simulink model "AB_switchtime_spline_real_time"  (R2025a)
settings: Solver=ode4  StartTime=0.0  StopTime=inf  FixedStep=1/500  RelTol=1e-3  EnableMultiTasking=on
InitFcn:
  | home = [0.45; 0; 0.49];
  | pick = [0.3; 0; 0.3];
  | place = [-0.25; -0.25; 0.01];
  | waypoints = ...
  | [pick, pick,place ,place ,home]' ;
undefined symbols (not defined in the file or in its folder): HIL, qc_get_step_size
libraries: quarc_library x19, simulink x2
(part 2 of 2)

== matlab function AB_switchtime_spline_real_time/objective position ==
  data: p input; gamma input; phi_optimal output; phi_prev input
function phi_optimal = qarmInverseKinematics_target(p, gamma, phi_prev)
%% QARM Inverse Kinematics (NaN-safe, limite saturée + workspace check)
% p        : position [x;y;z] en m
% gamma    : rotation poignet (rad)
% phi_prev : configuration précédente [4x1] en rad
% phi_optimal : configuration atteignable [4x1] rad

%% Paramètres du manipulateur
L1 = 0.1400; L2 = 0.3500; L3 = 0.0500; L4 = 0.2500; L5 = 0.1500;
beta = atan(L3/L2);
lambda1 = L1;
lambda2 = sqrt(L2^2 + L3^2);
lambda3 = L4 + L5;

%% Initialisation
theta = zeros(4,4);
phi   = zeros(4,4);

%% --- Calcul theta2 / theta3 ---
A = lambda2; 
C = -lambda3; 
H = lambda1 - p(3);

D1 = -sqrt(p(1)^2 + p(2)^2); 
D2 =  sqrt(p(1)^2 + p(2)^2);

F1 = (D1^2 + H^2 - A^2 - C^2)/(2*A);
F2 = (D2^2 + H^2 - A^2 - C^2)/(2*A);

% Solutions 1/2
if C^2 - F1^2 < 0
    warning('Position non atteignable pour solution 1/2 : saturation');
    theta(3,1) = sign(C)*pi/2;  
    theta(3,2) = sign(C)*pi/2;
else
    theta(3,1) = 2*atan2( C + sqrt(C^2 - F1^2), F1 );
    theta(3,2) = 2*atan2( C - sqrt(C^2 - F1^2), F1 );
end

% Solutions 3/4
if C^2 - F2^2 < 0
    warning('Position non atteignable pour solution 3/4 : saturation');
    theta(3,3) = sign(C)*pi/2;
    theta(3,4) = sign(C)*pi/2;
else
    theta(3,3) = 2*atan2( C + sqrt(C^2 - F2^2), F2 );
    theta(3,4) = 2*atan2( C - sqrt(C^2 - F2^2), F2 );
end

%% --- Calcul theta2 ---
for i = 1:4
    D = D1; 
    if i > 2
        D = D2;
    end
    M = A + C*sin(theta(3,i));
    N = -C*cos(theta(3,i));
    if abs(M) < 1e-6
        M = sign(M)*1e-6;
    end
    cos_term = (D*M + H*N)/(M^2 + N^2);
    sin_term = (H - N*cos_term)/M;
    theta(2,i) = atan2(sin_term, cos_term);
end

%% --- Calcul theta1 ---
for i = 1:4
    denom = lambda2*cos(theta(2,i)) - lambda3*sin(theta(2,i)+theta(3,i));
    if abs(denom) < 1e-6
        denom = sign(denom)*1e-6;
    end
    theta(1,i) = atan2(p(2)/denom, p(1)/denom);
end

%% --- Remap vers angles QARM ---
phi(1,:) = theta(1,:);
phi(2,:) = theta(2,:) - beta + pi/2;
phi(3,:) = theta(3,:) + beta;
phi(4,:) = gamma;
phi = mod(phi+pi, 2*pi) - pi; % normalisation [-pi,pi]

%% --- Saturation des limites articulaires ---
for i = 1:4
    phi(:,i) = saturate_joint_limits(phi(:,i));
end

%% --- Choix solution la plus proche de phi_prev dans le workspace ---
phi_optimal = phi_prev;     % par défaut: on reste où on est
best_norm   = inf;

for i = 1:4
    if ~isInsideWorkspace(phi(:,i))
        continue;           % solution rejetée: hors workspace
    end

    current_norm = norm(phi(:,i) - phi_prev);
    if current_norm < best_norm
        phi_optimal = phi(:,i);
        best_norm   = current_norm;
    end
end

if isinf(best_norm)
    warning('Aucune solution IK dans le workspace. On garde phi_prev.');
    phi_optimal = phi_prev;
end

end

%% --- Fonction de saturation ---
function phi_sat = saturate_joint_limits(phi)
limits = [
    -170  170;
    -80    80;
    -95    75;
    -160  160
]*pi/180;
phi_sat = phi;
for i = 1:4
    if phi(i) < limits(i,1), phi_sat(i) = limits(i,1); end
    if phi(i) > limits(i,2), phi_sat(i) = limits(i,2); end
end
end

%% --- Test de workspace via cinématique directe ---
function inside = isInsideWorkspace(phi)
    % Paramètres de l'enveloppe
    rMax = 0.8 * 0.78;      % rayon maximal autorisé (à ajuster)

    % Robot persistant pour la FK
    persistent robot eeName
    if isempty(robot)
        robot = loadrobot("quanserQArm", DataFormat="row");
        eeName = robot.BodyNames{end};
    end

    % Cinématique directe
    T = getTransform(robot, phi', eeName);   % phi' = row vector
    p = tform2trvec(T);                     % [x y z]

    x = p(1); y = p(2); z = p(3);
    r = norm(p);

    % 1) dedans la sphère
    % 2) pas dans le quadrant x<0 & z<0
    inside = (r < rMax) && ~((x < 0) && (z < 0));
end

== matlab function AB_switchtime_spline_real_time/Time_computation ==
  data: q0 input; T_min output size=1; q_end input
function T_min = T_min (q0, q_end)
    v_max = deg2rad([90 90 90 90]);
    T_vector = abs(q_end - q0) ./ v_max;
    T_min = max(T_vector(:)) * 1.2;
   
end

== matlab function AB_switchtime_spline_real_time/is_the_target_changed?1 ==
  data: p_obj input; final_p_obj output
function final_p_obj  = out_of_target(p_obj)
    eps_val = 1e-6;
    R_max = 0.7;

    norm_p = norm(p_obj);
    
    if norm_p > R_max
        final_p_obj = R_max * (p_obj / (norm_p + eps_val));
    else
        final_p_obj = p_obj;
    end
    
end

== matlab function AB_switchtime_spline_real_time/forward kinematics1 ==
  data: p3 output; R03 output; phi input; p4 output; R04 output; p_cam_0 output; p_obj_0 output; p_obj_cam input
function [p3, R03, p4, R04, p_cam_0,p_obj_0] = qarmForwardKinematics_target(phi,p_obj_cam)

%% QUANSER_ARM_FPK
% v 4.0 - 4th June 2020

% REFERENCE: 
% Chapter 3. Forward Kinematics
% Robot Dynamics and Control 
% Spong, Vidyasagar
% 1989

% INPUTS:
% phi     : Alternate joint angles vector 4 x 1

% OUTPUTS:
% p4      : End-effector frame {4} position vector expressed in base frame {0}
% R04     : rotation matrix from end-effector frame {4} to base frame {0}

%% Manipulator parameters:
L1 = 0.1400;
L2 = 0.3500;
L3 = 0.0500;
L4 = 0.2500;
L5 = 0.1500;

%% Alternate parameters
l1 = L1;
l2 = sqrt(L2^2 + L3^2);
l3 = L4 + L5;
beta = atan(L3/L2);

%% From phi space to theta space 
theta = phi;
theta(1) = phi(1);
theta(2) = phi(2) + beta - pi/2;
theta(3) = phi(3) - beta;
theta(4) = phi(4);

%% Transformation matrices for all frames:

% T{i-1}{i} = quanser_arm_DH(  a, alpha,  d,     theta );
        T01 = quanser_arm_DH(  0, -pi/2, l1,  theta(1) );
        T12 = quanser_arm_DH( l2,     0,  0,  theta(2) );
        T23 = quanser_arm_DH(  0, -pi/2,  0,  theta(3) );
        T34 = quanser_arm_DH(  0,     0, l3,  theta(4) );

        T02 = T01*T12;
        T03 = T02*T23;
        T04 = T03*T34;

%% Position of end-effector Transformation

% Extract the Position vector 
% p1   = T01(1:3,4);
% p2   = T02(1:3,4);
p3   = T03(1:3,4);
p4   = T04(1:3,4);

% Extract the Rotation matrix
% R01 = T01(1:3,1:3);
% R02 = T02(1:3,1:3);
R03 = T03(1:3,1:3);
R04 = T04(1:3,1:3);

d_tilde = 0.3; % distance entre P03 et la caméra (m)

% position de la caméra dans le frame de l'articulation 3
p_cam_3 = [0; 0; d_tilde]; 

% position de la caméra dans le frame global {0}
p_cam_0 = p3 + R03 * p_cam_3;

R_cam_3 = [ -1  0  0;
             0  1  0;
             0  0 -1 ];  % exemple si on inverse X et Z

R_cam_3 = [ 0  -1  0;
             1 0  0;
             0  0 1 ];  % exemple si on inverse X et Z

R_cam_0 = R03 * R_cam_3;  % rotation de la caméra dans le global

p_obj_0 = p_cam_0 + R_cam_0 * p_obj_cam;


end

function T = quanser_arm_DH(a,alpha,d,theta)

%% QUANSER_ARM_DH
% v 1.0 - 26th March 2019

% REFERENCE: 
% Chapter 3. Forward and Inverse Kinematics
% Robot Modeling and Control 
% Spong, Hutchinson, Vidyasagar
% 2006

% INPUTS:
% a       :   translation  : along : x_{i}   : from : z_{i-1} : to : z_{i}
% alpha   :      rotation  : about : x_{i}   : from : z_{i-1} : to : z_{i}
% d       :   translation  : along : z_{i-1} : from : x_{i-1} : to : x_{i}
% theta   :      rotation  : about : z_{i-1} : from : x_{i-1} : to : x_{i}
% NOTE: Standard DH Parameters

% OUTPUTS:
% T       : transformation                   : from :     {i} : to : {i-1}

%%
% Rotation Transformation about z axis by theta
T_R_z = [cos(theta) -sin(theta) 0 0;
         sin(theta)  cos(theta) 0 0;
                  0           0 1 0;
                  0           0 0 1];
     
% Translation Transformation along z axis by d
T_T_z = [1 0 0 0;
         0 1 0 0;
         0 0 1 d;
         0 0 0 1];

% Translation Transformation along x axis by a
T_T_x = [1 0 0 a;
         0 1 0 0;
         0 0 1 0;
         0 0 0 1];

% Rotation Transformation about x axis by alpha
T_R_x = [1          0           0 0;
         0 cos(alpha) -sin(alpha) 0;
         0 sin(alpha)  cos(alpha) 0;
         0          0           0 1];

% For a transformation FROM frame {i} TO frame {i-1}: A
T = T_R_z*T_T_z*T_T_x*T_R_x;

end

== matlab function AB_switchtime_spline_real_time/is_the_target_changed? ==
  data: p_target input; newTarget output; time output
function [newTarget, time]= Target_changed(p_target)

    persistent p_prev
    persistent T
        if isempty(p_prev)
            p_prev = zeros(size(p_target));
        end

        if isempty(T)
            T = 0.01;
        end
    
        %distance p_target and p_prev
        dp = p_target - p_prev;
        norm_dp = norm(dp);
   
        threshold = 0.05;   % [m]
    
        if norm_dp > threshold
            newTarget = 1;
            p_prev = p_target;
            T = 0.01;

               
        else
            newTarget = 0;
            T = T+0.01;
            %we don't switch

        
            
        end 
        time = T;
    
        
end

== matlab function AB_switchtime_spline_real_time/forward kinematics ==
  data: phi input; p4 output; R04 output
function [p4, R04] = qarmForwardKinematics(phi)

%% QUANSER_ARM_FPK
% v 4.0 - 4th June 2020

% REFERENCE: 
% Chapter 3. Forward Kinematics
% Robot Dynamics and Control 
% Spong, Vidyasagar
% 1989

% INPUTS:
% phi     : Alternate joint angles vector 4 x 1

% OUTPUTS:
% p4      : End-effector frame {4} position vector expressed in base frame {0}
% R04     : rotation matrix from end-effector frame {4} to base frame {0}

%% Manipulator parameters:
L1 = 0.1400;
L2 = 0.3500;
L3 = 0.0500;
L4 = 0.2500;
L5 = 0.1500;

%% Alternate parameters
l1 = L1;
l2 = sqrt(L2^2 + L3^2);
l3 = L4 + L5;
beta = atan(L3/L2);

%% From phi space to theta space 
theta = phi;
theta(1) = phi(1);
theta(2) = phi(2) + beta - pi/2;
theta(3) = phi(3) - beta;
theta(4) = phi(4);

%% Transformation matrices for all frames:

% T{i-1}{i} = quanser_arm_DH(  a, alpha,  d,     theta );
        T01 = quanser_arm_DH(  0, -pi/2, l1,  theta(1) );
        T12 = quanser_arm_DH( l2,     0,  0,  theta(2) );
        T23 = quanser_arm_DH(  0, -pi/2,  0,  theta(3) );
        T34 = quanser_arm_DH(  0,     0, l3,  theta(4) );

        T02 = T01*T12;
        T03 = T02*T23;
        T04 = T03*T34;

%% Position of end-effector Transformation

% Extract the Position vector 
% p1   = T01(1:3,4);
% p2   = T02(1:3,4);
% p3   = T03(1:3,4);
p4   = T04(1:3,4);

% Extract the Rotation matrix
% R01 = T01(1:3,1:3);
% R02 = T02(1:3,1:3);
% R03 = T03(1:3,1:3);
R04 = T04(1:3,1:3);

end

function T = quanser_arm_DH(a,alpha,d,theta)

%% QUANSER_ARM_DH
% v 1.0 - 26th March 2019

% REFERENCE: 
% Chapter 3. Forward and Inverse Kinematics
% Robot Modeling and Control 
% Spong, Hutchinson, Vidyasagar
% 2006

% INPUTS:
% a       :   translation  : along : x_{i}   : from : z_{i-1} : to : z_{i}
% alpha   :      rotation  : about : x_{i}   : from : z_{i-1} : to : z_{i}
% d       :   translation  : along : z_{i-1} : from : x_{i-1} : to : x_{i}
% theta   :      rotation  : about : z_{i-1} : from : x_{i-1} : to : x_{i}
% NOTE: Standard DH Parameters

% OUTPUTS:
% T       : transformation                   : from :     {i} : to : {i-1}

%%
% Rotation Transformation about z axis by theta
T_R_z = [cos(theta) -sin(theta) 0 0;
         sin(theta)  cos(theta) 0 0;
                  0           0 1 0;
                  0           0 0 1];
     
% Translation Transformation along z axis by d
T_T_z = [1 0 0 0;
         0 1 0 0;
         0 0 1 d;
         0 0 0 1];

% Translation Transformation along x axis by a
T_T_x = [1 0 0 a;
         0 1 0 0;
         0 0 1 0;
         0 0 0 1];

% Rotation Transformation about x axis by alpha
T_R_x = [1          0           0 0;
         0 cos(alpha) -sin(alpha) 0;
         0 sin(alpha)  cos(alpha) 0;
         0          0           0 1];

% For a transformation FROM frame {i} TO frame {i-1}: A
T = T_R_z*T_T_z*T_T_x*T_R_x;

end

== matlab function AB_switchtime_spline_real_time/target_phi ==
  data: coeffs input; q output; t input
function q = evalCubic4(coeffs, t)
% coeffs: 4x4, righe = [a0;a1;a2;a3], colonne = giunti
% t: scalare
% q: 4x1

    a0 = coeffs(1, :).';  % 4x1
    a1 = coeffs(2, :).';
    a2 = coeffs(3, :).';
    a3 = coeffs(4, :).';

    q = a0 + a1*t + a2*(t^2) + a3*(t^3);
end

== matlab function AB_switchtime_spline_real_time/differential kinematics ==
  data: phi input; J output
function J   = qarmDifferentialKinematics(phi)

%% QUANSER_ARM_FDK
% v 1.0 - 13th August 2020

% REFERENCE: 
% Chapter 5. Velocity Kinematics
% Robot Dynamics and Control 
% Spong, Vidyasagar
% 1989

% INPUTS:
% phi     : Alternate joint angles vector 4 x 1

% OUTPUTS:
% p4      : End-effector frame {4} position vector expressed in base frame {0}
% R04     : rotation matrix from end-effector frame {4} to base frame {0}

%% Manipulator parameters:
L1 = 0.1400;
L2 = 0.3500;
L3 = 0.0500;
L4 = 0.2500;
L5 = 0.1500;

%% Alternate parameters
l1 = L1;
l2 = sqrt(L2^2 + L3^2);
l3 = L4 + L5;
beta = atan(L3/L2);

%% From phi space to theta space 
theta = phi;
theta(1) = phi(1);
theta(2) = phi(2) + beta - pi/2;
theta(3) = phi(3) - beta;
theta(4) = phi(4);

%% Precompute sines and cosines
c1 = cos(theta(1)); s1 = sin(theta(1));
c2 = cos(theta(2)); s2 = sin(theta(2));
c23 = cos(theta(2) + theta(3)); s23 = sin(theta(2) + theta(3));

%% Jacobian term definition:

J = eye(4);
J(1,1) = -l2 * s1 * c2 + l3 * s1 * s23;
J(1,2) = -l2 * c1 * s2 - l3 * c1 * c23;
J(1,3) = -l3 * c1 * c23;
J(1,4) = 0;

J(2,1) =  l2 * c1 * c2 - l3 * c1 * s23;
J(2,2) = -l2 * s1 * s2 - l3 * s1 * c23;
J(2,3) = -l3 * s1 * c23;
J(2,4) = 0;

J(3,1) =  0;
J(3,2) = -l2 * c2 + l3 * s23;
J(3,3) =  l3 * s23;
J(3,4) = 0;

J(4,1) =  0;
J(4,2) =  0;
J(4,3) =  0;
J(4,4) =  1;

end

== matlab function AB_switchtime_spline_real_time/forward kinematics - measurement ==
  data: phi input; p4 output; R04 output
function [p4, R04] = qarmForwardKinematics(phi)

%% QUANSER_ARM_FPK
% v 4.0 - 4th June 2020

% REFERENCE: 
% Chapter 3. Forward Kinematics
% Robot Dynamics and Control 
% Spong, Vidyasagar
% 1989

% INPUTS:
% phi     : Alternate joint angles vector 4 x 1

% OUTPUTS:
% p4      : End-effector frame {4} position vector expressed in base frame {0}
% R04     : rotation matrix from end-effector frame {4} to base frame {0}

%% Manipulator parameters:
L1 = 0.1400;
L2 = 0.3500;
L3 = 0.0500;
L4 = 0.2500;
L5 = 0.1500;

%% Alternate parameters
l1 = L1;
l2 = sqrt(L2^2 + L3^2);
l3 = L4 + L5;
beta = atan(L3/L2);

%% From phi space to theta space 
theta = phi;
theta(1) = phi(1);
theta(2) = phi(2) + beta - pi/2;
theta(3) = phi(3) - beta;
theta(4) = phi(4);

%% Transformation matrices for all frames:

% T{i-1}{i} = quanser_arm_DH(  a, alpha,  d,     theta );
        T01 = quanser_arm_DH(  0, -pi/2, l1,  theta(1) );
        T12 = quanser_arm_DH( l2,     0,  0,  theta(2) );
        T23 = quanser_arm_DH(  0, -pi/2,  0,  theta(3) );
        T34 = quanser_arm_DH(  0,     0, l3,  theta(4) );

        T02 = T01*T12;
        T03 = T02*T23;
        T04 = T03*T34;

%% Position of end-effector Transformation

% Extract the Position vector 
% p1   = T01(1:3,4);
% p2   = T02(1:3,4);
% p3   = T03(1:3,4);
p4   = T04(1:3,4);

% Extract the Rotation matrix
% R01 = T01(1:3,1:3);
% R02 = T02(1:3,1:3);
% R03 = T03(1:3,1:3);
R04 = T04(1:3,1:3);

end

function T = quanser_arm_DH(a,alpha,d,theta)

%% QUANSER_ARM_DH
% v 1.0 - 26th March 2019

% REFERENCE: 
% Chapter 3. Forward and Inverse Kinematics
% Robot Modeling and Control 
% Spong, Hutchinson, Vidyasagar
% 2006

% INPUTS:
% a       :   translation  : along : x_{i}   : from : z_{i-1} : to : z_{i}
% alpha   :      rotation  : about : x_{i}   : from : z_{i-1} : to : z_{i}
% d       :   translation  : along : z_{i-1} : from : x_{i-1} : to : x_{i}
% theta   :      rotation  : about : z_{i-1} : from : x_{i-1} : to : x_{i}
% NOTE: Standard DH Parameters

% OUTPUTS:
% T       : transformation                   : from :     {i} : to : {i-1}

%%
% Rotation Transformation about z axis by theta
T_R_z = [cos(theta) -sin(theta) 0 0;
         sin(theta)  cos(theta) 0 0;
                  0           0 1 0;
                  0           0 0 1];
     
% Translation Transformation along z axis by d
T_T_z = [1 0 0 0;
         0 1 0 0;
         0 0 1 d;
         0 0 0 1];

% Translation Transformation along x axis by a
T_T_x = [1 0 0 a;
         0 1 0 0;
         0 0 1 0;
         0 0 0 1];

% Rotation Transformation about x axis by alpha
T_R_x = [1          0           0 0;
         0 cos(alpha) -sin(alpha) 0;
         0 sin(alpha)  cos(alpha) 0;
         0          0           0 1];

% For a transformation FROM frame {i} TO frame {i-1}: A
T = T_R_z*T_T_z*T_T_x*T_R_x;

end

== matlab function AB_switchtime_spline_real_time/forward kinematics3 ==
  data: phi input; p4 output; R04 output
function [p4, R04] = qarmForwardKinematics(phi)

%% QUANSER_ARM_FPK
% v 4.0 - 4th June 2020

% REFERENCE: 
% Chapter 3. Forward Kinematics
% Robot Dynamics and Control 
% Spong, Vidyasagar
% 1989

% INPUTS:
% phi     : Alternate joint angles vector 4 x 1

% OUTPUTS:
% p4      : End-effector frame {4} position vector expressed in base frame {0}
% R04     : rotation matrix from end-effector frame {4} to base frame {0}

%% Manipulator parameters:
L1 = 0.1400;
L2 = 0.3500;
L3 = 0.0500;
L4 = 0.2500;
L5 = 0.1500;

%% Alternate parameters
l1 = L1;
l2 = sqrt(L2^2 + L3^2);
l3 = L4 + L5;
beta = atan(L3/L2);

%% From phi space to theta space 
theta = phi;
theta(1) = phi(1);
theta(2) = phi(2) + beta - pi/2;
theta(3) = phi(3) - beta;
theta(4) = phi(4);

%% Transformation matrices for all frames:

% T{i-1}{i} = quanser_arm_DH(  a, alpha,  d,     theta );
        T01 = quanser_arm_DH(  0, -pi/2, l1,  theta(1) );
        T12 = quanser_arm_DH( l2,     0,  0,  theta(2) );
        T23 = quanser_arm_DH(  0, -pi/2,  0,  theta(3) );
        T34 = quanser_arm_DH(  0,     0, l3,  theta(4) );

        T02 = T01*T12;
        T03 = T02*T23;
        T04 = T03*T34;

%% Position of end-effector Transformation

% Extract the Position vector 
% p1   = T01(1:3,4);
% p2   = T02(1:3,4);
% p3   = T03(1:3,4);
p4   = T04(1:3,4);

% Extract the Rotation matrix
% R01 = T01(1:3,1:3);
% R02 = T02(1:3,1:3);
% R03 = T03(1:3,1:3);
R04 = T04(1:3,1:3);

end

function T = quanser_arm_DH(a,alpha,d,theta)

%% QUANSER_ARM_DH
% v 1.0 - 26th March 2019

% REFERENCE: 
% Chapter 3. Forward and Inverse Kinematics
% Robot Modeling and Control 
% Spong, Hutchinson, Vidyasagar
% 2006

% INPUTS:
% a       :   translation  : along : x_{i}   : from : z_{i-1} : to : z_{i}
% alpha   :      rotation  : about : x_{i}   : from : z_{i-1} : to : z_{i}
% d       :   translation  : along : z_{i-1} : from : x_{i-1} : to : x_{i}
% theta   :      rotation  : about : z_{i-1} : from : x_{i-1} : to : x_{i}
% NOTE: Standard DH Parameters

% OUTPUTS:
% T       : transformation                   : from :     {i} : to : {i-1}

%%
% Rotation Transformation about z axis by theta
T_R_z = [cos(theta) -sin(theta) 0 0;
         sin(theta)  cos(theta) 0 0;
                  0           0 1 0;
                  0           0 0 1];
     
% Translation Transformation along z axis by d
T_T_z = [1 0 0 0;
         0 1 0 0;
         0 0 1 d;
         0 0 0 1];

% Translation Transformation along x axis by a
T_T_x = [1 0 0 a;
         0 1 0 0;
         0 0 1 0;
         0 0 0 1];

% Rotation Transformation about x axis by alpha
T_R_x = [1          0           0 0;
         0 cos(alpha) -sin(alpha) 0;
         0 sin(alpha)  cos(alpha) 0;
         0          0           0 1];

% For a transformation FROM frame {i} TO frame {i-1}: A
T = T_R_z*T_T_z*T_T_x*T_R_x;

end

== matlab function AB_switchtime_spline_real_time/forward kinematics - setpoint ==
  data: phi input; p4 output; R04 output
function [p4, R04] = qarmForwardKinematics(phi)

%% QUANSER_ARM_FPK
% v 4.0 - 4th June 2020

% REFERENCE: 
% Chapter 3. Forward Kinematics
% Robot Dynamics and Control 
% Spong, Vidyasagar
% 1989

% INPUTS:
% phi     : Alternate joint angles vector 4 x 1

% OUTPUTS:
% p4      : End-effector frame {4} position vector expressed in base frame {0}
% R04     : rotation matrix from end-effector frame {4} to base frame {0}

%% Manipulator parameters:
L1 = 0.1400;
L2 = 0.3500;
L3 = 0.0500;
L4 = 0.2500;
L5 = 0.1500;

%% Alternate parameters
l1 = L1;
l2 = sqrt(L2^2 + L3^2);
l3 = L4 + L5;
beta = atan(L3/L2);

%% From phi space to theta space 
theta = phi;
theta(1) = phi(1);
theta(2) = phi(2) + beta - pi/2;
theta(3) = phi(3) - beta;
theta(4) = phi(4);

%% Transformation matrices for all frames:

% T{i-1}{i} = quanser_arm_DH(  a, alpha,  d,     theta );
        T01 = quanser_arm_DH(  0, -pi/2, l1,  theta(1) );
        T12 = quanser_arm_DH( l2,     0,  0,  theta(2) );
        T23 = quanser_arm_DH(  0, -pi/2,  0,  theta(3) );
        T34 = quanser_arm_DH(  0,     0, l3,  theta(4) );

        T02 = T01*T12;
        T03 = T02*T23;
        T04 = T03*T34;

%% Position of end-effector Transformation

% Extract the Position vector 
% p1   = T01(1:3,4);
% p2   = T02(1:3,4);
% p3   = T03(1:3,4);
p4   = T04(1:3,4);

% Extract the Rotation matrix
% R01 = T01(1:3,1:3);
% R02 = T02(1:3,1:3);
% R03 = T03(1:3,1:3);
R04 = T04(1:3,1:3);

end

function T = quanser_arm_DH(a,alpha,d,theta)

%% QUANSER_ARM_DH
% v 1.0 - 26th March 2019

% REFERENCE: 
% Chapter 3. Forward and Inverse Kinematics
% Robot Modeling and Control 
% Spong, Hutchinson, Vidyasagar
% 2006

% INPUTS:
% a       :   translation  : along : x_{i}   : from : z_{i-1} : to : z_{i}
% alpha   :      rotation  : about : x_{i}   : from : z_{i-1} : to : z_{i}
% d       :   translation  : along : z_{i-1} : from : x_{i-1} : to : x_{i}
% theta   :      rotation  : about : z_{i-1} : from : x_{i-1} : to : x_{i}
% NOTE: Standard DH Parameters

% OUTPUTS:
% T       : transformation                   : from :     {i} : to : {i-1}

%%
% Rotation Transformation about z axis by theta
T_R_z = [cos(theta) -sin(theta) 0 0;
         sin(theta)  cos(theta) 0 0;
                  0           0 1 0;
                  0           0 0 1];
     
% Translation Transformation along z axis by d
T_T_z = [1 0 0 0;
         0 1 0 0;
         0 0 1 d;
         0 0 0 1];

% Translation Transformation along x axis by a
T_T_x = [1 0 0 a;
         0 1 0 0;
         0 0 1 0;
         0 0 0 1];

% Rotation Transformation about x axis by alpha
T_R_x = [1          0           0 0;
         0 cos(alpha) -sin(alpha) 0;
         0 sin(alpha)  cos(alpha) 0;
         0          0           0 1];

% For a transformation FROM frame {i} TO frame {i-1}: A
T = T_R_z*T_T_z*T_T_x*T_R_x;

end
